simulink model "Lego_robot_control_udp"  (R2019b)
settings: Solver=ode3  StartTime=0.0  StopTime=inf  RelTol=1e-3  EnableMultiTasking=on
InitFcn:
  | K = [0.4175    0.5498]; %Velocity Control Gains
undefined symbols (not defined in the file): DiscIntNeverNeededParam
libraries: legoev3lib x13, simulink x2, simulink_extras x1
CloseFcn:
  | clear K
settings Model: SimulationMode=external  ExtModeTrigDuration=2  Creator=The MathWorks, Inc.  LastModifiedBy=shiqihang
settings SolverCC: PositivePriorityOrder=on
settings DataIOCC: LimitDataPoints=on  SaveFormat=Array  ReturnWorkspaceOutputs=off
settings OptimizationCC: LifeSpan=Inf  MaxStackSize=64
settings DebuggingCC: UnderspecifiedInitializationDetection=Classic  MergeDetectMultiDrivingBlocksExec=none  IntegerOverflowMsg=none  AllowSymbolicDim=off  SFUnexpectedBacktrackingDiag=warning  SFNoUnconditionalDefaultTransitionDiag=warning  SFExecutionAtInitializationDiag=none  IntegerSaturationMsg=none  ArithmeticOperatorsInVariantConditions=warning
settings HardwareCC: ProdBitPerPointer=32  ProdBitPerSizeT=32  ProdBitPerPtrDiffT=32  ProdLargestAtomicInteger=Long  ProdWordSize=32  ProdHWDeviceType=ARM Compatible->ARM 9  UseEmbeddedCoderFeatures=off  UseSimulinkCoderFeatures=off
settings ModelReferenceCC: PropagateSignalLabelsOutOfModel=off
settings SFSimCC: SimUseLocalCustomCode=off  CustomCodeUndefinedFunction=UseInterfaceOnly
settings RTWCC: SystemTargetFile=ert.tlc  HardwareBoard=LEGO MINDSTORMS EV3  TemplateMakefile=ert_default_tmf  RTWVerbose=off  RTWUseLocalCustomCode=off  Toolchain=Sourcery G++ Lite v2009q3  BuildConfiguration=Faster Runs
settings CodeAppCC: ForceParamTrailComments=on  OperatorAnnotations=on  MangleLength=10  StateflowObjectComments=on  MATLABSourceComments=on
settings ERTTargetCC: MultiwordLength=2048  ERTCustomFileBanners=off  SupportContinuousTime=on  SupportNonInlinedSFcns=on  RemoveResetFunc=off  ModelStepFunctionPrototypeControlCompliant=off  ExtMode=on  ExtModeMexArgs='192.168.1.3' 0 17725  ERTSrcFileBannerTemplate=codertarget_code_template.cgt  ERTHdrFileBannerTemplate=codertarget_code_template.cgt  ERTDataSrcFileTemplate=codertarget_code_template.cgt  ERTDataHdrFileTemplate=codertarget_code_template.cgt
settings ConfigComp: CovMetricSettings=dw  CovHtmlReporting=on  CovSaveCumulativeToWorkspaceVar=on  CovSaveSingleToWorkspaceVar=on  CovExternalEMLEnable=off  CovSFcnEnable=off

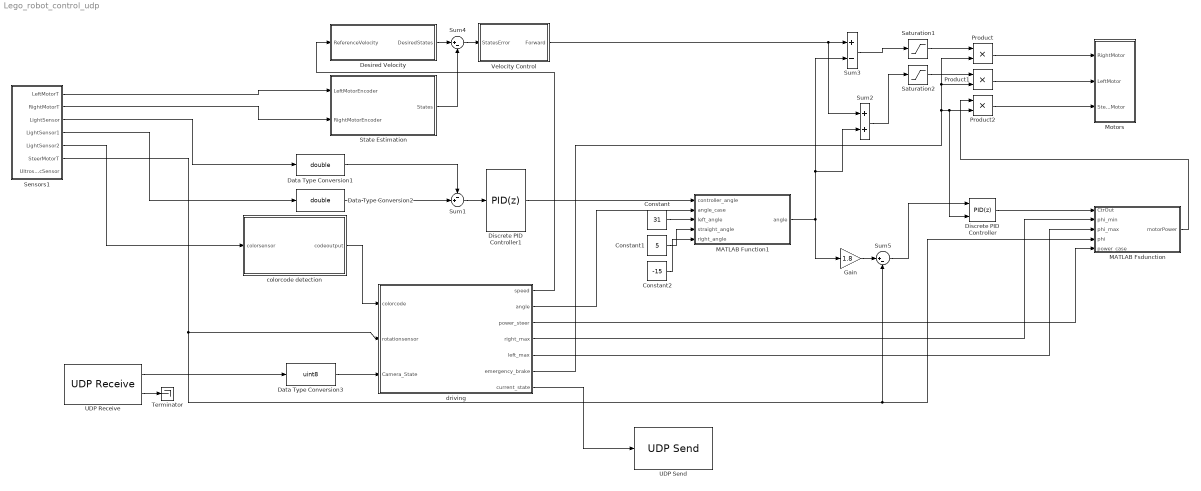
== system Lego_robot_control_udp ==
  Constant : Constant  Value=31
  Constant1 : Constant  Value=5
  Constant2 : Constant  Value=-15
  Data Type Conversion1 : DataTypeConversion  OutDataTypeStr=double
  Data Type Conversion2 : DataTypeConversion  OutDataTypeStr=double
  Data Type Conversion3 : DataTypeConversion  OutDataTypeStr=uint8
  Desired Velocity : Subsystem
  Discrete PID Controller : simulink/Continuous/PID Controller  Controller=PID  Form=Parallel  TimeDomain=Discrete-time  SampleTime=-1  IntegratorMethod=Forward Euler  FilterMethod=Forward Euler  ControllerParametersSource=internal  P=0.9  I=1  D=0.04  UseFilter=on  N=100  TunerSelectOption=Transfer Function Based (PID Tuner App)  InitialConditionSource=internal  InitialConditionForIntegrator=0  InitialConditionForFilter=0  DifferentiatorICPrevScaledInput=0  ExternalReset=either  TrackingMode=off  Kt=1  LimitOutput=on  UpperSaturationLimit=100  LowerSaturationLimit=-100  LinearizeAsGain=off  AntiWindupMode=none  Kb=1  POutMin=[]  POutMax=[]  IOutMin=[]  IOutMax=[]  DOutMin=[]  DOutMax=[]  NOutMin=[]  NOutMax=[]  SumOutMin=[]  SumOutMax=[]  SaturationOutMin=[]  SaturationOutMax=[]  PParamMin=[]  PParamMax=[]  IParamMin=[]  IParamMax=[]  DParamMin=[]  DParamMax=[]  NParamMin=[]  NParamMax=[]  KbParamMin=[]  KbParamMax=[]  KtParamMin=[]  KtParamMax=[]  KbOutMin=[]  KbOutMax=[]  KtOutMin=[]  KtOutMax=[]  IntegratorOutMin=[]  IntegratorOutMax=[]  FilterOutMin=[]  FilterOutMax=[]  SumI1OutMin=[]  SumI1OutMax=[]  SumI2OutMin=[]  SumI2OutMax=[]  SumI3OutMin=[]  SumI3OutMax=[]  SumI4OutMin=[]  SumI4OutMax=[]  SumDOutMin=[]  SumDOutMax=[]  DifferentiatorOutMin=[]  DifferentiatorOutMax=[]  FilterDiffOutCoefMin=[]  FilterDiffOutCoefMax=[]  ReciprocalOutMin=[]  ReciprocalOutMax=[]  SumDenOutMin=[]  SumDenOutMax=[]  SumNumOutMin=[]  SumNumOutMax=[]  DivideOutMin=[]  DivideOutMax=[]  IntegratorContinuousStateAttributes=''  IntegratorStateMustResolveToSignalObject=off  IntegratorRTWStateStorageClass=Auto  FilterContinuousStateAttributes=''  FilterStateMustResolveToSignalObject=off  FilterRTWStateStorageClass=Auto  ParallelPVariant=InternalParameters  IdealPVariant=Disabled  IVariant=InternalParameters  DVariant=InternalParameters  IntegratorVariant=Discrete  SatVariant=Enabled  AWVariant=Passthrough  PCopyVariant=Disabled  TRVariant=Disabled  FdbkBlocksVariant=Forward  IdealPFdbkVariant=Disabled  SatFdbkVariant=Disabled  DerivativeFilterVariant=ForwardEulerFilter  NVariant=InternalParameters  NCopyVariant=Disabled  FilterICVariant=InternalICsFilter  IntegratorICVariant=InternalICs  ExternalResetVariant=ExternalReset  TRSumVariant=Passthrough  SumFdbkVariant=Disabled  SumVariant=Sum_PID
  Discrete PID Controller1 : simulink/Continuous/PID Controller  Controller=PID  Form=Parallel  TimeDomain=Discrete-time  SampleTime=-1  IntegratorMethod=Forward Euler  FilterMethod=Forward Euler  ControllerParametersSource=internal  P=2.85  I=0.1  D=0.05  UseFilter=on  N=100  TunerSelectOption=Transfer Function Based (PID Tuner App)  InitialConditionSource=internal  InitialConditionForIntegrator=0  InitialConditionForFilter=0  DifferentiatorICPrevScaledInput=0  ExternalReset=none  TrackingMode=off  Kt=1  LimitOutput=on  UpperSaturationLimit=100  LowerSaturationLimit=-100  LinearizeAsGain=off  AntiWindupMode=none  Kb=1  POutMin=[]  POutMax=[]  IOutMin=[]  IOutMax=[]  DOutMin=[]  DOutMax=[]  NOutMin=[]  NOutMax=[]  SumOutMin=[]  SumOutMax=[]  SaturationOutMin=[]  SaturationOutMax=[]  PParamMin=[]  PParamMax=[]  IParamMin=[]  IParamMax=[]  DParamMin=[]  DParamMax=[]  NParamMin=[]  NParamMax=[]  KbParamMin=[]  KbParamMax=[]  KtParamMin=[]  KtParamMax=[]  KbOutMin=[]  KbOutMax=[]  KtOutMin=[]  KtOutMax=[]  IntegratorOutMin=[]  IntegratorOutMax=[]  FilterOutMin=[]  FilterOutMax=[]  SumI1OutMin=[]  SumI1OutMax=[]  SumI2OutMin=[]  SumI2OutMax=[]  SumI3OutMin=[]  SumI3OutMax=[]  SumI4OutMin=[]  SumI4OutMax=[]  SumDOutMin=[]  SumDOutMax=[]  DifferentiatorOutMin=[]  DifferentiatorOutMax=[]  FilterDiffOutCoefMin=[]  FilterDiffOutCoefMax=[]  ReciprocalOutMin=[]  ReciprocalOutMax=[]  SumDenOutMin=[]  SumDenOutMax=[]  SumNumOutMin=[]  SumNumOutMax=[]  DivideOutMin=[]  DivideOutMax=[]  IntegratorContinuousStateAttributes=''  IntegratorStateMustResolveToSignalObject=off  IntegratorRTWStateStorageClass=Auto  FilterContinuousStateAttributes=''  FilterStateMustResolveToSignalObject=off  FilterRTWStateStorageClass=Auto  ParallelPVariant=InternalParameters  IdealPVariant=Disabled  IVariant=InternalParameters  DVariant=InternalParameters  IntegratorVariant=Discrete  SatVariant=Enabled  AWVariant=Passthrough  PCopyVariant=Disabled  TRVariant=Disabled  FdbkBlocksVariant=Forward  IdealPFdbkVariant=Disabled  SatFdbkVariant=Disabled  DerivativeFilterVariant=ForwardEulerFilter  NVariant=InternalParameters  NCopyVariant=Disabled  FilterICVariant=InternalICsFilter  IntegratorICVariant=InternalICs  ExternalResetVariant=Disabled  TRSumVariant=Passthrough  SumFdbkVariant=Disabled  SumVariant=Sum_PID
  Gain : Gain  Gain=1.8
  MATLAB Fsdunction : MATLAB Function  TreatAsAtomicUnit=on
  MATLAB Function1 : MATLAB Function  TreatAsAtomicUnit=on
  Motors : Subsystem
  Product : Product
  Product1 : Product
  Product2 : Product
  Saturation1 : Saturate  UpperLimit=0  LowerLimit=-inf
  Saturation2 : Saturate  UpperLimit=0  LowerLimit=-inf
  Sensors1 : Subsystem
  State Estimation : Subsystem
  Sum1 : Sum  Inputs=-+|
  Sum2 : Sum
  Sum3 : Sum  Inputs=+-
  Sum4 : Sum  Inputs=|+-
  Sum5 : Sum  Inputs=|+-
  Terminator : Terminator
  UDP Receive : legoev3lib/UDP Receive  localURL='0.0.0.0'  localPort=25000  remoteURL='0.0.0.0'  remotePort=-1  recvBufferSize=8192  signalDatatype=uint8  dims=1  isVarSize=off  showBlockingTime=off  blockingTime=0  sampletime=0.004  blockPlatform=LEGO EV3
      settings: SourceProductName=Simulink Support Package for LEGO MINDSTORMS EV3 Hardware  SourceProductBaseCode=LEGOEV3
  UDP Send : legoev3lib/UDP Send  remoteURL='192.168.1.2'  remotePort=25001  localURL='0.0.0.0'  localPortSource=Automatically determine  localPort=2048  sampletime=-1  blockPlatform=LEGO EV3  separateLengthPort=0
      settings: SourceProductName=Simulink Support Package for LEGO MINDSTORMS EV3 Hardware  SourceProductBaseCode=LEGOEV3
  Velocity Control : Subsystem
  colorcode detection : Stateflow chart  TreatAsAtomicUnit=on
  driving : Stateflow chart  TreatAsAtomicUnit=on
  wires:
  Sensors1/4(LightSensor1) -> Data Type Conversion2/1
  MATLAB Function1/1(angle) -> Gain/1, Sum2/2, Sum3/2
  Sum1/1 -> Discrete PID Controller1/1
  State Estimation/1(States) -> Sum4/2
  driving/1(speed) -> Desired Velocity/1(ReferenceVelocity)
  Desired Velocity/1(DesiredStates) -> Sum4/1
  Velocity Control/1(Forward) -> Sum3/1, Sum2/1
  Sum4/1 -> Velocity Control/1(StatesError)
  Sensors1/3(LightSensor) -> Data Type Conversion1/1
  Sensors1/1(LeftMotorT) -> State Estimation/1(LeftMotorEncoder)
  Sensors1/2(RightMotorT) -> State Estimation/2(RightMotorEncoder)
  Sum3/1 -> Saturation1/1
  Sum2/1 -> Saturation2/1
  Sensors1/6(SteerMotorT) -> Sum5/2, MATLAB Fsdunction/4(phi), driving/2(rotationsensor)
  MATLAB Fsdunction/1(motorPower) -> Product2/1
  Gain/1 -> Sum5/1
  Sum5/1 -> Discrete PID Controller/1
  Discrete PID Controller/1 -> MATLAB Fsdunction/1(CtrOut)
  Sensors1/5(LightSensor2) -> colorcode detection/1(colorsensor)
  colorcode detection/1(codeoutput) -> driving/1(colorcode)
  driving/4(right_max) -> MATLAB Fsdunction/2(phi_min)
  Discrete PID Controller1/1 -> MATLAB Function1/1(controller_angle)
  driving/2(angle) -> MATLAB Function1/2(angle_case)
  driving/5(left_max) -> MATLAB Fsdunction/3(phi_max)
  driving/3(power_steer) -> MATLAB Fsdunction/5(power_case)
  Constant/1 -> MATLAB Function1/3(left_angle)
  Constant1/1 -> MATLAB Function1/4(straight_angle)
  Data Type Conversion1/1 -> Sum1/1
  Data Type Conversion2/1 -> Sum1/2
  Saturation1/1 -> Product/1
  Saturation2/1 -> Product1/1
  Constant2/1 -> MATLAB Function1/5(right_angle)
  Data Type Conversion3/1 -> driving/3(Camera_State)
  driving/6(emergency_brake) -> Product/2, Product1/2, Discrete PID Controller/2, Product2/2
  Product/1 -> Motors/1(RightMotor)
  Product1/1 -> Motors/2(LeftMotor)
  Product2/1 -> Motors/3(SteerMotor)
  UDP Receive/1 -> Data Type Conversion3/1
  UDP Receive/2 -> Terminator/1
  driving/7(current_state) -> UDP Send/1

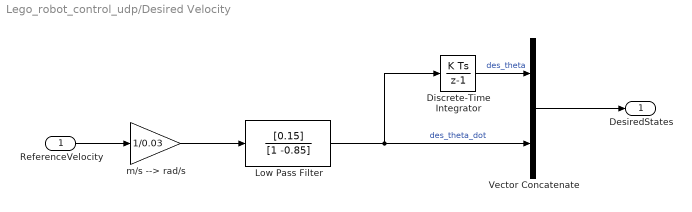
== system Lego_robot_control_udp/Desired Velocity ==
  ReferenceVelocity : Inport
  Discrete-Time Integrator : DiscreteIntegrator  SampleTime=-1  ICPrevOutput=DiscIntNeverNeededParam  ICPrevScaledInput=DiscIntNeverNeededParam
  Low Pass Filter : DiscreteFilter  Numerator=[0.15]  Denominator=[1 -0.85]
  Vector Concatenate : Concatenate
  m/s --> rad/s : Gain  Gain=1/0.03
  DesiredStates : Outport  VectorParamsAs1DForOutWhenUnconnected=off
  wires:
  Vector Concatenate/1 -> DesiredStates/1
  ReferenceVelocity/1 -> m/s --> rad/s/1
  m/s --> rad/s/1 -> Low Pass Filter/1
  Discrete-Time Integrator/1 -> Vector Concatenate/1  "des_theta"
  Low Pass Filter/1 -> Discrete-Time Integrator/1, Vector Concatenate/2  "des_theta_dot"

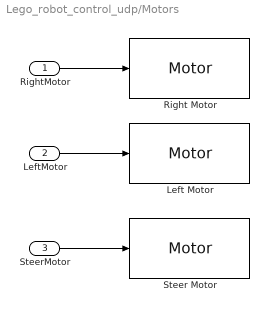
== system Lego_robot_control_udp/Motors ==
  RightMotor : Inport
  LeftMotor : Inport  Port=2
  SteerMotor : Inport  Port=3
  " Left Motor" : legoev3lib/Motor  sportNumber=A  sstopAction=Brake
  Right Motor : legoev3lib/Motor  sportNumber=C  sstopAction=Brake
  Steer Motor : legoev3lib/Motor  sportNumber=B  sstopAction=Brake
  wires:
  RightMotor/1 -> Right Motor/1
  LeftMotor/1 -> " Left Motor"/1
  SteerMotor/1 -> Steer Motor/1

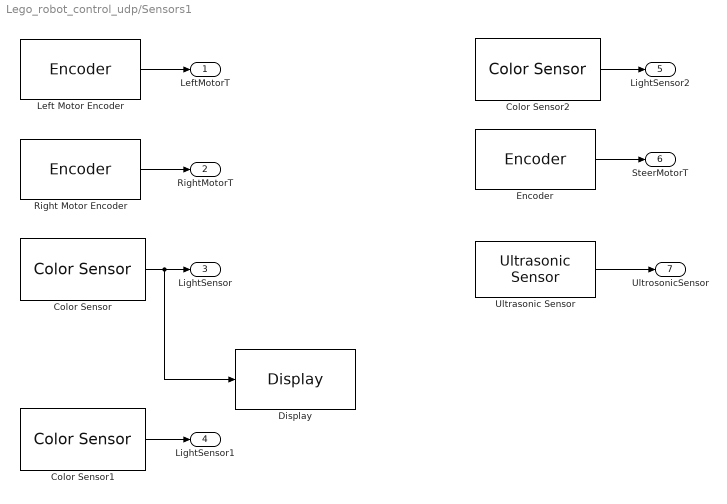
== system Lego_robot_control_udp/Sensors1 ==
  Color Sensor : legoev3lib/Color Sensor  portNumber=1  mode=Reflected light intensity  sampleTime=0.004
      settings: SourceProductName=Simulink Support Package for LEGO MINDSTORMS EV3 Hardware  SourceProductBaseCode=LEGOEV3
  Color Sensor1 : legoev3lib/Color Sensor  portNumber=3  mode=Reflected light intensity  sampleTime=0.004
      settings: SourceProductName=Simulink Support Package for LEGO MINDSTORMS EV3 Hardware  SourceProductBaseCode=LEGOEV3
  Color Sensor2 : legoev3lib/Color Sensor  portNumber=2  mode=Color  sampleTime=0.004
      settings: SourceProductName=Simulink Support Package for LEGO MINDSTORMS EV3 Hardware  SourceProductBaseCode=LEGOEV3
  Display : legoev3lib/Display  slcdStr=light  slcdLine=1  slcdFormat=Decimal
      settings: SourceProductName=Simulink Support Package for LEGO MINDSTORMS EV3 Hardware  SourceProductBaseCode=LEGOEV3
  Encoder : legoev3lib/Encoder  portNumber=B  opMode=No reset  sampleTime=0.004
      settings: SourceProductName=Simulink Support Package for LEGO MINDSTORMS EV3 Hardware  SourceProductBaseCode=LEGOEV3
  Left Motor Encoder : legoev3lib/Encoder  portNumber=A  opMode=No reset  sampleTime=0.004
      settings: SourceProductName=Simulink Support Package for LEGO MINDSTORMS EV3 Hardware  SourceProductBaseCode=LEGOEV3
  Right Motor Encoder : legoev3lib/Encoder  portNumber=C  opMode=No reset  sampleTime=0.004
      settings: SourceProductName=Simulink Support Package for LEGO MINDSTORMS EV3 Hardware  SourceProductBaseCode=LEGOEV3
  Ultrasonic Sensor : legoev3lib/Ultrasonic Sensor  PortNumber=4  sampleTime=0.004
      settings: SourceProductName=Simulink Support Package for LEGO MINDSTORMS EV3 Hardware  SourceProductBaseCode=LEGOEV3
  LeftMotorT : Outport  VectorParamsAs1DForOutWhenUnconnected=off
  RightMotorT : Outport  Port=2  VectorParamsAs1DForOutWhenUnconnected=off
  LightSensor : Outport  Port=3  VectorParamsAs1DForOutWhenUnconnected=off
  LightSensor1 : Outport  Port=4  VectorParamsAs1DForOutWhenUnconnected=off
  LightSensor2 : Outport  Port=5  VectorParamsAs1DForOutWhenUnconnected=off
  SteerMotorT : Outport  Port=6  VectorParamsAs1DForOutWhenUnconnected=off
  UltrosonicSensor : Outport  Port=7  VectorParamsAs1DForOutWhenUnconnected=off
  wires:
  Left Motor Encoder/1 -> LeftMotorT/1
  Right Motor Encoder/1 -> RightMotorT/1
  Color Sensor/1 -> Display/1, LightSensor/1
  Color Sensor1/1 -> LightSensor1/1
  Color Sensor2/1 -> LightSensor2/1
  Encoder/1 -> SteerMotorT/1
  Ultrasonic Sensor/1 -> UltrosonicSensor/1

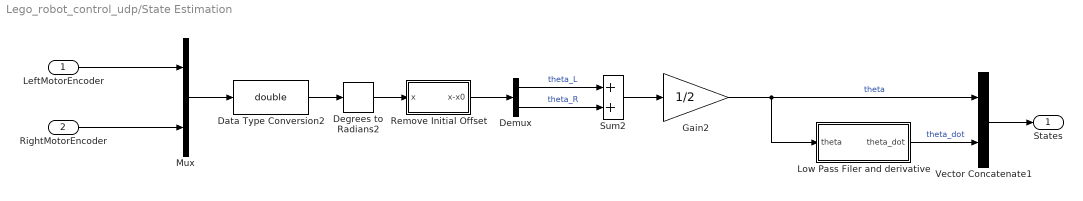
== system Lego_robot_control_udp/State Estimation ==
  LeftMotorEncoder : Inport
  RightMotorEncoder : Inport  Port=2
  Data Type Conversion2 : DataTypeConversion  OutDataTypeStr=double
  Degrees to Radians2 : simulink_extras/Transformations/Degrees to Radians
  Demux : Demux  Outputs=2
  Gain2 : Gain  Gain=1/2
  Low Pass Filer and derivative : Subsystem
  Mux : Mux  Inputs=2
  Remove Initial Offset : Subsystem
  Sum2 : Sum
  Vector Concatenate1 : Concatenate
  States : Outport  VectorParamsAs1DForOutWhenUnconnected=off
  wires:
  Remove Initial Offset/1(x-x0) -> Demux/1
  LeftMotorEncoder/1 -> Mux/1
  RightMotorEncoder/1 -> Mux/2
  Demux/1 -> Sum2/1  "theta_L"
  Demux/2 -> Sum2/2  "theta_R"
  Vector Concatenate1/1 -> States/1
  Gain2/1 -> Low Pass Filer and derivative/1(theta), Vector Concatenate1/1  "theta"
  Sum2/1 -> Gain2/1
  Data Type Conversion2/1 -> Degrees to Radians2/1
  Degrees to Radians2/1 -> Remove Initial Offset/1(x)
  Mux/1 -> Data Type Conversion2/1
  Low Pass Filer and derivative/1(theta_dot) -> Vector Concatenate1/2  "theta_dot"

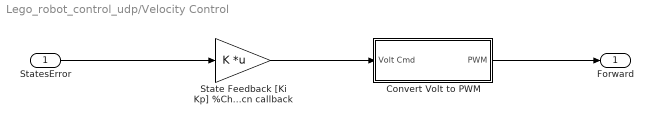
== system Lego_robot_control_udp/Velocity Control ==
  StatesError : Inport
  " State Feedback [Ki Kp] %Change these values in the model's InitFcn callback" : Gain  Gain=K  Multiplication=Matrix(K*u)
  Convert Volt to PWM : Subsystem
  Forward : Outport  VectorParamsAs1DForOutWhenUnconnected=off
  wires:
  StatesError/1 -> " State Feedback [Ki Kp] %Change these values in the model's InitFcn callback"/1
  " State Feedback [Ki Kp] %Change these values in the model's InitFcn callback"/1 -> Convert Volt to PWM/1(Volt Cmd)
  Convert Volt to PWM/1(PWM) -> Forward/1

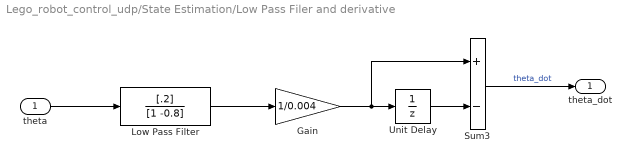
== system Lego_robot_control_udp/State Estimation/Low Pass Filer and derivative ==
  theta : Inport
  Gain : Gain  Gain=1/0.004
  Low Pass Filter : DiscreteFilter  Numerator=[.2]  Denominator=[1 -0.8]
  Sum3 : Sum  Inputs=+-
  Unit Delay : UnitDelay  SampleTime=-1  HasFrameUpgradeWarning=on
  theta_dot : Outport  VectorParamsAs1DForOutWhenUnconnected=off
  wires:
  Unit Delay/1 -> Sum3/2
  Gain/1 -> Unit Delay/1, Sum3/1
  Sum3/1 -> theta_dot/1  "theta_dot"
  Low Pass Filter/1 -> Gain/1
  theta/1 -> Low Pass Filter/1

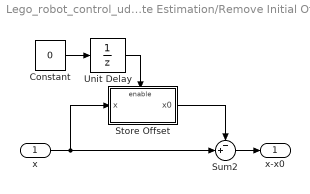
== system Lego_robot_control_udp/State Estimation/Remove Initial Offset ==
  x : Inport
  Constant : Constant  Value=0  OutDataTypeStr=boolean
  Store Offset : Subsystem  TreatAsAtomicUnit=on
  Sum2 : Sum  Inputs=-+|
  Unit Delay : UnitDelay  InitialCondition=1  SampleTime=-1  HasFrameUpgradeWarning=on
  x-x0 : Outport  VectorParamsAs1DForOutWhenUnconnected=off
  wires:
  Sum2/1 -> x-x0/1
  Unit Delay/1 -> Store Offset/Enable
  Constant/1 -> Unit Delay/1
  Store Offset/1(x0) -> Sum2/1
  x/1 -> Store Offset/1(x), Sum2/2

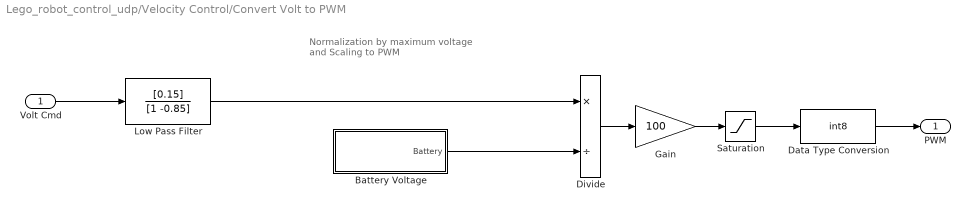
== system Lego_robot_control_udp/Velocity Control/Convert Volt to PWM ==
  note: Normalization by maximum voltage
      | and
      | Scaling to PWM
  Volt Cmd : Inport
  Battery Voltage : Subsystem
  Data Type Conversion : DataTypeConversion  OutDataTypeStr=int8
  Divide : Product  Inputs=*/
  Gain : Gain  Gain=100
  Low Pass Filter : DiscreteFilter  Numerator=[0.15]  Denominator=[1 -0.85]
  Saturation : Saturate  UpperLimit=100  LowerLimit=-100
  PWM : Outport  VectorParamsAs1DForOutWhenUnconnected=off
  wires:
  Data Type Conversion/1 -> PWM/1
  Saturation/1 -> Data Type Conversion/1
  Volt Cmd/1 -> Low Pass Filter/1
  Gain/1 -> Saturation/1
  Divide/1 -> Gain/1
  Low Pass Filter/1 -> Divide/1
  Battery Voltage/1(Battery) -> Divide/2

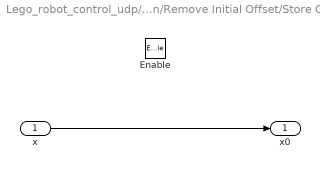
== system Lego_robot_control_udp/State Estimation/Remove Initial Offset/Store Offset ==
  x : Inport
  Enable : EnablePort
  x0 : Outport  InitialOutput=0  VectorParamsAs1DForOutWhenUnconnected=off
  wires:
  x/1 -> x0/1

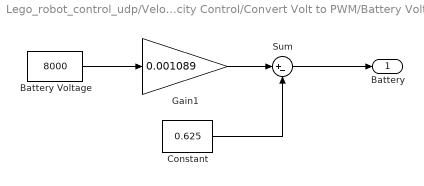
== system Lego_robot_control_udp/Velocity Control/Convert Volt to PWM/Battery Voltage ==
  Battery Voltage : Constant  Value=8000
  Constant : Constant  Value=0.625
  Gain1 : Gain  Gain=0.001089
  Sum : Sum  Inputs=|+-
  Battery : Outport  VectorParamsAs1DForOutWhenUnconnected=off
  wires:
  Sum/1 -> Battery/1
  Battery Voltage/1 -> Gain1/1
  Constant/1 -> Sum/2
  Gain1/1 -> Sum/1

== matlab function Lego_robot_control_udp/MATLAB Fsdunction ==
  data: CtrOut input; phi_min input; phi_max input; phi input; motorPower output; power_case input
function motorPower = func1(CtrOut, phi_min,phi_max,phi,power_case)
if (phi > phi_max) && (CtrOut > 0)
    motorPower = 0;
elseif (phi < phi_min) && (CtrOut < 0)
    motorPower = 0;
elseif power_case < 99   %case for calibration
    motorPower = power_case;
else
    motorPower = CtrOut;
end
end

== stateflow chart Lego_robot_control_udp/driving ==
  state start
    entry:
    speed = 0;
    angle=0;
    right_max = -80;
    left_max = 80;
    emergency_brake=1;
    current_state = 0;
  state cross_decision
    entry:
    current_state = 2;
    state four_cross
      entry:
      decision = rand;
    state three_cross_ls
      entry:
      decision = rand;
    state three_cross_lr
      entry:
      decision = rand;
    state three_cross_rs
      entry:
      decision = rand;
    four_cross -> (junction 121) [order 3]
    four_cross -> (junction 118) [order 2] : [0.333<=decision<0.666]
    four_cross -> (junction 115) [order 1] : [decision <0.333]
    three_cross_ls -> (junction 115) [order 1] : [decision<1]
    three_cross_ls -> (junction 118) [order 2]
    three_cross_lr -> (junction 115) [order 1] : [decision<0.5]
    three_cross_lr -> (junction 121) [order 2]
    three_cross_rs -> (junction 118) [order 1] : [decision<0.5]
    three_cross_rs -> (junction 121) [order 2]
  state linefollow
    during:
    speed=-0.2;
    angle =  0;
    power_steer = 100;
    current_state = 1;
  state turn_left
    entry:
    %angle = 2;
    current_state=5;
    speed=0;
    power_steer=0;
    state start_go_straight1
      during:
      speed=-0.2;
      power_steer=100;
      angle=1;
      emergency_brake=1;
    state Wait
      entry:
      turn_finish=0;
      emergency_brake=0;
    state Finish
      entry:
      turn_finish=1;
      emergency_brake=1;
    (default) -> turn_left.Wait
    turn_left.Wait -> start_go_straight1 : after(2,sec)[Camera_State==3]
    start_go_straight1 -> turn_left.Finish : after(1.4,sec)
  state turn_right
    entry:
    %angle = 3;
    current_state=3;
    angle=0;
    speed=0;
    power_steer=0;
    state Wait
      entry:
      turn_finish=0;
      emergency_brake=0;
    state start_turn_right
      during:
      emergency_brake=1;
      speed=-0.4;
      power_steer=100;
      angle=3;
    state Finish
      entry:
      turn_finish=1;
      emergency_brake=1;
    (default) -> turn_right.Wait
    turn_right.Wait -> start_turn_right : [Camera_State==1]
    start_turn_right -> turn_right.Finish : after(1,sec)
  state drive_straight
    entry:
    %angle = 1;
    angle=0;
    power_steer=0;
    speed=0;
    current_state = 4;
    state Wait
      entry:
      turn_finish=0;
      emergency_brake=0;
    state start_drive_straight
      during:
      speed=-0.4;
      power_steer=100;
      angle=1;
      emergency_brake=1;
    state Finish
      entry:
      turn_finish=1;
      emergency_brake=1;
    (default) -> drive_straight.Wait
    drive_straight.Wait -> start_drive_straight : [Camera_State==2]
    start_drive_straight -> drive_straight.Finish : after(0.01,sec)
  (default) -> start
  (junction 121) -> turn_right : [colorcode==5]
  (junction 118) -> drive_straight : [colorcode==5]
  (junction 115) -> turn_left : [colorcode==5]
  linefollow -> four_cross [order 1] : [colorcode==4]
  start -> linefollow
  linefollow -> three_cross_ls [order 4] : [colorcode==3]
  linefollow -> three_cross_lr [order 3] : [colorcode==2]
  linefollow -> three_cross_rs [order 2] : [colorcode==1]
  turn_right -> linefollow : [turn_finish==1]
  turn_left -> linefollow : [turn_finish==1]
  drive_straight -> linefollow : [turn_finish==1]
  data: colorcode input double; speed output double; angle output double; rotationsensor input int32; power_steer output double; right_max output int32; decision local double; left_max output int32; middle local int32; past local int32; Camera_State input uint8; emergency_brake output; turn_finish local; current_state output uint8

== stateflow chart Lego_robot_control_udp/colorcode detection ==
  state output2
    entry:
    codeoutput = 1;
  state output1
    entry:
    codeoutput = 5;
  state start
    entry:
    last_color = 0;
    codeoutput = 0;
  state detect
  state output
    entry:
    codeoutput = 3;
  state safe
    entry:
    last_color = colorsensor;
    codeoutput=0;
  (junction 32) -> output2 [order 3] : [(last_color==5)&&(colorsensor==4) ]
  output2 -> safe
  (default) -> start
  (junction 32) -> output1 [order 2] : [(last_color==4)&&(colorsensor==5) ]
  output1 -> safe
  start -> detect
  (junction 32) -> safe [order 4]
  detect -> (junction 32) : [last_color ~= colorsensor]
  (junction 32) -> output [order 1] : [((last_color==4)&&(colorsensor==2))||((last_color==3)&&(colorsensor==5)) ]
  output -> safe
  safe -> detect
  data: colorsensor input uint8; codeoutput output; last_color local uint8

== matlab function Lego_robot_control_udp/MATLAB Function1 ==
  data: controller_angle input; angle_case input; angle output; left_angle input; straight_angle input; right_angle input
function angle = fcn(controller_angle,angle_case,left_angle,straight_angle,right_angle)

if angle_case == 1
    angle = straight_angle;
elseif angle_case == 2
    angle = left_angle;
elseif angle_case == 3
    angle = right_angle;
else
    angle = controller_angle;
end
end
